simulink model "Mo_hinh_DC_motor_2vong_dk"  (R2019a)
settings: Solver=VariableStepAuto  StartTime=0.0  StopTime=0.1  RelTol=1e-3
values from neighbouring files (symbols this model uses):
  J = 0.36    [Thong_so_dong_co_1_chieu.m]
  K1oc = 0.1    [Thong_so_dong_co_1_chieu.m]
  K2p = K1oc/(4*Tcp*K2*K2oc)    (= 351.858377202)    [Thong_so_dong_co_1_chieu.m]
  Kcp = 10    [Thong_so_dong_co_1_chieu.m]
  Ke = 30*(Ua-Ra*Ia)/(pi*n)    (= 0.339713042931)    [Thong_so_dong_co_1_chieu.m]
  Ki = Kp/T2    [Thong_so_dong_co_1_chieu.m]
  Km = M/Ia    (= 0.255784729969)    [Thong_so_dong_co_1_chieu.m]
  Kp = (T2*Ke)/(2*T1*Kcp*K1oc)    [Thong_so_dong_co_1_chieu.m]
  Ra = 0.585    [Thong_so_dong_co_1_chieu.m]    (also in mTinh_Toan_Thong_so.m = 0.2305)
  Ta = La/Ra    (= 0.0427522435656)    [Thong_so_dong_co_1_chieu.m]
  Tcp = 0.002    [Thong_so_dong_co_1_chieu.m]
libraries: powerlib x1
settings Model: Creator=Admin  LastModifiedBy=Admin

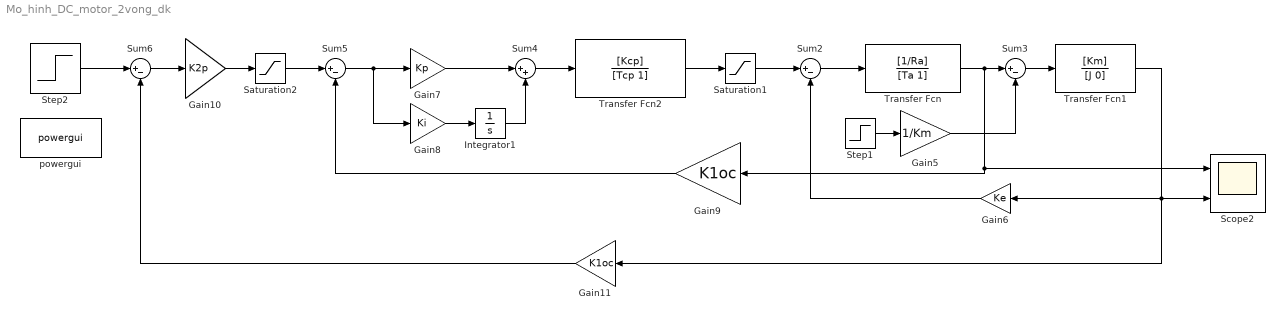
== system Mo_hinh_DC_motor_2vong_dk ==
  Gain10 : Gain  Gain=K2p
  Gain11 : Gain  Gain=K1oc
  Gain5 : Gain  Gain=1/Km
  Gain6 : Gain  Gain=Ke
  Gain7 : Gain  Gain=Kp
  Gain8 : Gain  Gain=Ki
  Gain9 : Gain  Gain=K1oc
  Integrator1 : Integrator
  Saturation1 : Saturate  UpperLimit=110  LowerLimit=-110
  Saturation2 : Saturate  UpperLimit=1.68  LowerLimit=-1.68
  Scope2 : Scope  NumInputPorts=2
  Step1 : Step  Time=0.6  After=0.1  SampleTime=0
  Step2 : Step  Time=0  After=0.05  SampleTime=0
  Sum{2..3,5..6} (4 alike) : Sum  Inputs=|+-
  Sum4 : Sum  Inputs=|++
  Transfer Fcn : TransferFcn  Numerator=[1/Ra]  Denominator=[Ta 1]
  Transfer Fcn1 : TransferFcn  Numerator=[Km]  Denominator=[J 0]
  Transfer Fcn2 : TransferFcn  Numerator=[Kcp]  Denominator=[Tcp 1]
  powergui : powerlib/powergui  Priority=1  SimulationMode=Continuous  SampleTime=50e-6  frequency=60  Iterations=50  frequencyindice=60  Pbase=100e6  ErrMax=1e-4  UnitsV=kV  UnitsW=MW  buscounter=0  FunctionMessages=off  echomessages=off  EnableUseOfTLC=off  CurrentSourceSwitches=off  DisableSnubberDevices=off  DisableRonSwitches=off  DisableVfSwitches=off  DisplayEquations=off  AutomaticDiscreteSolvers=off  SolverType=Tustin/Backward Euler (TBE)  Interpol=off  ExternalGateDelay=off  methode=off  Ts=100  x0status=blocks  SPID=on  SwTol=0  HookPort=off  NonlinearTolerance=0  nMaxIteration=15  ContinueOnMaxIteration=off  RestoreLinks=warning  ResistiveCurrentMeasurement=off  Frange=[0:2:500]  Ylog=off  Xlog=on  ShowGrid=off  save=off  variable=ZData  structure=0  ZoomFFT=off  StartTime=0.0  cycles=1  DisplayStyle=1  fundamental=60  FreqAxis=off  MaxFrequency=1000  frequencyindicesteady=1  RmsSteady=1  display=off
      settings: SourceProductName=Simscape Electrical
  wires:
  Saturation1/1 -> Sum2/1
  Transfer Fcn2/1 -> Saturation1/1
  Sum2/1 -> Transfer Fcn/1
  Gain6/1 -> Sum2/2
  Integrator1/1 -> Sum4/2
  Step2/1 -> Sum6/1
  Gain7/1 -> Sum4/1
  Sum3/1 -> Transfer Fcn1/1
  Step1/1 -> Gain5/1
  Saturation2/1 -> Sum5/1
  Gain11/1 -> Sum6/2
  Sum6/1 -> Gain10/1
  Gain10/1 -> Saturation2/1
  Gain8/1 -> Integrator1/1
  Gain9/1 -> Sum5/2
  Transfer Fcn/1 -> Gain9/1, Scope2/1, Sum3/1
  Gain5/1 -> Sum3/2
  Transfer Fcn1/1 -> Scope2/2, Gain11/1, Gain6/1
  Sum4/1 -> Transfer Fcn2/1
  Sum5/1 -> Gain8/1, Gain7/1
